simulink model "FireFighter_original"  (R2014a)
settings: Solver=ode45  StartTime=0.0  StopTime=150  RelTol=1e-3
undefined symbols (not defined in the file): DiscIntNeverNeededParam, sigbuilder_block
libraries: simulink x68
(part 1 of 6)
settings Model: NumberOfSteps=200  Creator=rima  LastModifiedBy=rima
settings DataIOCC: InspectSignalLogs=on
settings OptimizationCC: ExpressionDepthLimit=2147483647
settings DebuggingCC: UnderspecifiedInitializationDetection=Classic  SolverPrmCheckMsg=none  StateNameClashWarn=warning

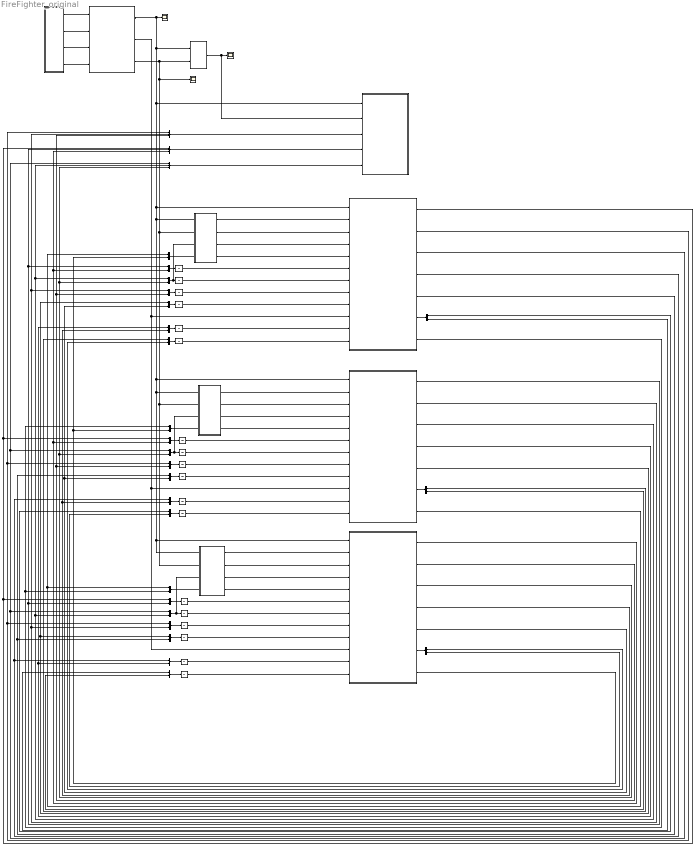
== system FireFighter_original ==
  Demux : Demux  Outputs=2
  Demux1 : Demux  Outputs=2
  Demux2 : Demux  Outputs=2
  FF_Signals : Subsystem
  FF_Signals1 : Subsystem
  FF_Signals2 : Subsystem
  FF_Signals4 : Subsystem
  FireFighter : Stateflow chart  TreatAsAtomicUnit=on
  Helicopter1 : Stateflow chart  TreatAsAtomicUnit=on
  Helicopter2 : Stateflow chart  TreatAsAtomicUnit=on
  Helicopter3 : Stateflow chart  TreatAsAtomicUnit=on
  Inaccuracy : Subsystem
  Leader : Stateflow chart  TreatAsAtomicUnit=on
  Mux{,1,3..7,9..17,20..22,27..28} (21 alike) : Mux  Inputs=2
  Mux18 : Mux  Inputs=3
  Mux19 : Mux  Inputs=3
  Mux2 : Mux  Inputs=3
  Scope1 : Scope
      settings: SaveName=ScopeData10
  Scope11 : Scope
      settings: SaveName=ScopeData37
  Scope2 : Scope
      settings: YMin=-2.5e+12  YMax=2.5e+11  SaveName=ScopeData14
  Unit Delay{,1..14,21..23} (18 alike) : UnitDelay
  wires:
  FF_Signals/1(conn) -> FireFighter/1(ffConn)
  FF_Signals/2(Hconn) -> FireFighter/2(ffHconn)
  Mux2/1 -> Leader/3(HFFPoss)
  Mux1/1 -> FF_Signals1/3(Hpos_inits), Unit Delay2/1
  Mux3/1 -> Unit Delay1/1
  Mux4/1 -> Unit Delay/1
  FireFighter/2(ffMID) -> Helicopter3/10(MID), Helicopter2/10(MID), Helicopter1/10(MID)
  Mux9/1 -> FF_Signals4/3(Hpos_inits), Unit Delay7/1
  Mux10/1 -> Unit Delay6/1
  Mux11/1 -> Unit Delay5/1
  Mux12/1 -> FF_Signals2/3(Hpos_inits), Unit Delay12/1
  Mux13/1 -> Unit Delay11/1
  Mux14/1 -> Unit Delay10/1
  Mux15/1 -> Unit Delay13/1
  Helicopter2/2(HFFPos) -> Mux2/2, Mux17/1, Mux15/2
  Helicopter1/2(HFFPos) -> Mux2/1, Mux16/1, Mux15/1
  Helicopter3/2(HFFPos) -> Mux2/3, Mux17/2, Mux16/2
  Mux16/1 -> Unit Delay8/1
  Mux17/1 -> Unit Delay3/1
  Helicopter1/5(Search_Out) -> Mux11/1, Mux14/2
  Helicopter2/5(Search_Out) -> Mux14/1, Mux4/1
  Helicopter3/5(Search_Out) -> Mux4/2, Mux11/2
  Helicopter3/1(HID) -> Mux18/3, Mux3/2, Mux10/2
  Helicopter1/1(HID) -> Mux18/1, Mux10/1, Mux13/1
  Helicopter2/1(HID) -> Mux18/2, Mux3/1, Mux13/2
  Helicopter2/3(HPos) -> Mux19/2, Mux1/1, Mux12/2
  Helicopter1/3(HPos) -> Mux19/1, Mux9/1, Mux12/1
  Helicopter3/3(HPos) -> Mux19/3, Mux1/2, Mux9/2
  Mux18/1 -> Leader/4(HIDs)
  Mux19/1 -> Leader/5(HPoss)
  Unit Delay5/1 -> Helicopter2/9(Search_In)
  Unit Delay6/1 -> Helicopter2/6(OHIDs)
  Unit Delay7/1 -> Helicopter2/7(OHPoss)
  Unit Delay8/1 -> Helicopter2/8(OHFFPos)
  Unit Delay10/1 -> Helicopter3/9(Search_In)
  Unit Delay11/1 -> Helicopter3/6(OHIDs)
  Unit Delay12/1 -> Helicopter3/7(OHPoss)
  Unit Delay13/1 -> Helicopter3/8(OHFFPos)
  FF_Signals/4(Activate) -> FireFighter/4(ffActivate)
  Mux5/1 -> Unit Delay4/1
  Helicopter3/4(Signal_Out) -> Mux6/2, Mux5/2
  Mux6/1 -> Unit Delay9/1
  Helicopter1/4(Signal_Out) -> Mux6/1, Mux7/1
  Mux7/1 -> Unit Delay14/1
  Helicopter2/4(Signal_Out) -> Mux7/2, Mux5/1
  Unit Delay9/1 -> Helicopter2/11(Signal_In)
  Unit Delay/1 -> Helicopter1/9(Search_In)
  Unit Delay1/1 -> Helicopter1/6(OHIDs)
  Unit Delay2/1 -> Helicopter1/7(OHPoss)
  Unit Delay3/1 -> Helicopter1/8(OHFFPos)
  Unit Delay4/1 -> Helicopter1/11(Signal_In)
  Helicopter1/6(Signal_Reply_Out) -> Demux/1
  Mux/1 -> Unit Delay21/1
  Mux27/1 -> Unit Delay22/1
  Helicopter2/6(Signal_Reply_Out) -> Demux1/1
  Mux28/1 -> Unit Delay23/1
  Helicopter3/6(Signal_Reply_Out) -> Demux2/1
  Demux1/1 -> Mux/1
  Demux2/1 -> Mux/2
  Demux/1 -> Mux27/1
  Demux2/2 -> Mux27/2
  Demux/2 -> Mux28/1
  Demux1/2 -> Mux28/2
  Unit Delay22/1 -> Helicopter2/12(Signal_Reply_In)
  Unit Delay23/1 -> Helicopter3/12(Signal_Reply_In)
  Unit Delay21/1 -> Helicopter1/12(Signal_Reply_In)
  Unit Delay14/1 -> Helicopter3/11(Signal_In)
  FF_Signals/3(FFPos_Out) -> FireFighter/3(ffPos_In)
  FireFighter/3(ffHold) -> Scope11/1, FF_Signals2/2(hold), FF_Signals4/2(hold), FF_Signals1/2(hold), Inaccuracy/2(hold)
  Inaccuracy/1(result) -> Scope2/1, Leader/2(FFPosInacc)
  FF_Signals1/1(HPos_Out) -> Helicopter1/2(HPos_In)
  FF_Signals1/4(SWITCH) -> Helicopter1/5(SWITCH)
  FF_Signals1/2(FFPos_inacc) -> Helicopter1/3(FFPosInacc)
  FireFighter/1(ffPos) -> Scope1/1, Helicopter2/1(FFPos), Helicopter3/1(FFPos), FF_Signals2/1(pos_init), FF_Signals4/1(pos_init), FF_Signals1/1(pos_init), Helicopter1/1(FFPos), Leader/1(FFPos_In), Inaccuracy/1(pos_init)
  FF_Signals4/1(HPos_Out) -> Helicopter2/2(HPos_In)
  FF_Signals4/4(SWITCH) -> Helicopter2/5(SWITCH)
  FF_Signals4/2(FFPos_inacc) -> Helicopter2/3(FFPosInacc)
  FF_Signals2/1(HPos_Out) -> Helicopter3/2(HPos_In)
  FF_Signals2/4(SWITCH) -> Helicopter3/5(SWITCH)
  FF_Signals2/2(FFPos_inacc) -> Helicopter3/3(FFPosInacc)
  FF_Signals1/3(HsInacc) -> Helicopter1/4(HsPosInacc)
  Mux20/1 -> FF_Signals1/4(holds)
  Helicopter2/7(hold) -> Mux20/1, Mux22/1
  Helicopter3/7(hold) -> Mux20/2, Mux21/2
  FF_Signals4/3(HsInacc) -> Helicopter2/4(HsPosInacc)
  Mux21/1 -> FF_Signals4/4(holds)
  Mux22/1 -> FF_Signals2/4(holds)
  Helicopter1/7(hold) -> Mux21/1, Mux22/2
  FF_Signals2/3(HsInacc) -> Helicopter3/4(HsPosInacc)

== system FireFighter_original/FF_Signals ==
  Environment : Subsystem
  FireFighter : Subsystem
  Helicopter Signal : Subsystem  Tag=STV Subsys  LoadFcn=sigbuilder_block('load');  StartFcn=sigbuilder_block('start');  StopFcn=sigbuilder_block('stop');  ClipboardFcn=sigbuilder_block('clipboard');  mask(Sigbuilder block){}
      mask help: Simulink:masks:SigbuilderBlock_MD
      mask init:
      | if ~strcmp(get_param(bdroot(gcbh),'SimulationStatus'),'stopped') tuvar = sigbuilder_block('maskInit'); end
      settings: CopyFcn=sigbuilder_block('copy');  DeleteFcn=sigbuilder_block('delete');  ModelCloseFcn=sigbuilder_block('modelClose');  PreSaveFcn=sigbuilder_block('preSave');  PauseFcn=sigbuilder_block('pause');  ContinueFcn=sigbuilder_block('continue');  NameChangeFcn=sigbuilder_block('namechange');  OpenFcn=sigbuilder_block('open',[451.5 315 606.75 510 ]);  CloseFcn=sigbuilder_block('close');
      mask Display: plot(0, 0, 100, 100,[2, 2, 32, 32, 2], [68, 8, 8, 68, 68],[32, 2], [38, 38], [32, 19, 2],[53, 60, 44], [32, 17, 17, 2],[16, 16, 31, 31]);txt = getActiveGroup(gcbh);text(2, 100, txt,'verticalAlignment', 'top');
  Mux : Mux
  Mux1 : Mux  Inputs=3
  START THE MESSION : Subsystem  Tag=STV Subsys  LoadFcn=sigbuilder_block('load');  StartFcn=sigbuilder_block('start');  StopFcn=sigbuilder_block('stop');  ClipboardFcn=sigbuilder_block('clipboard');  mask(Sigbuilder block){}
      mask help: Simulink:masks:SigbuilderBlock_MD
      mask init:
      | if ~strcmp(get_param(bdroot(gcbh),'SimulationStatus'),'stopped') tuvar = sigbuilder_block('maskInit'); end
      settings: CopyFcn=sigbuilder_block('copy');  DeleteFcn=sigbuilder_block('delete');  ModelCloseFcn=sigbuilder_block('modelClose');  PreSaveFcn=sigbuilder_block('preSave');  PauseFcn=sigbuilder_block('pause');  ContinueFcn=sigbuilder_block('continue');  NameChangeFcn=sigbuilder_block('namechange');  OpenFcn=sigbuilder_block('open',[76.5 537.75 597.75 240 ]);  CloseFcn=sigbuilder_block('close');
      mask Display: plot(0, 0, 100, 100,[2, 2, 32, 32, 2], [68, 8, 8, 68, 68],[32, 2], [38, 38], [32, 19, 2],[53, 60, 44], [32, 17, 17, 2],[16, 16, 31, 31]);txt = getActiveGroup(gcbh);text(2, 100, txt,'verticalAlignment', 'top');
  Scope : Scope
      settings: YMin=1.38778e-17  YMax=0.45  SaveName=ScopeData11
  Scope1 : Scope
      settings: SaveName=ScopeData47
  conn : Outport
  Hconn : Outport  Port=2
  FFPos_Out : Outport  Port=3
  Activate : Outport  Port=4
  wires:
  Environment/1(pos) -> FireFighter/1(pos), Scope/1, FFPos_Out/1
  FireFighter/1(gas) -> Environment/1(gas)
  FireFighter/2(brake) -> Environment/2(brake)
  Helicopter Signal/1(CONN) -> Mux/1, conn/1
  Helicopter Signal/2(HCONN1) -> Mux1/1, Mux/2
  Helicopter Signal/4(HCONN3) -> Mux/4, Mux1/3
  START THE MESSION/1(ACTIVATE) -> Activate/1
  Helicopter Signal/3(HCONN2) -> Mux/3, Mux1/2
  Mux/1 -> Scope1/1
  Mux1/1 -> Hconn/1

== system FireFighter_original/FF_Signals1 ==
  pos_init : Inport
  hold : Inport  Port=2
  Hpos_inits : Inport  Port=3
  holds : Inport  Port=4
  Demux{,1..3} (4 alike) : Demux  Outputs=2
  Environment1 : Subsystem
  FireFighter1 : Subsystem
  Inaccuracy : Subsystem
  Inaccuracy1 : Subsystem
  Inaccuracy2 : Subsystem
  Mux : Mux
  START THE MESSION2 : Subsystem  Tag=STV Subsys  LoadFcn=sigbuilder_block('load');  StartFcn=sigbuilder_block('start');  StopFcn=sigbuilder_block('stop');  ClipboardFcn=sigbuilder_block('clipboard');  mask(Sigbuilder block){}
      mask help: Simulink:masks:SigbuilderBlock_MD
      mask init:
      | if ~strcmp(get_param(bdroot(gcbh),'SimulationStatus'),'stopped') tuvar = sigbuilder_block('maskInit'); end
      settings: CopyFcn=sigbuilder_block('copy');  DeleteFcn=sigbuilder_block('delete');  ModelCloseFcn=sigbuilder_block('modelClose');  PreSaveFcn=sigbuilder_block('preSave');  PauseFcn=sigbuilder_block('pause');  ContinueFcn=sigbuilder_block('continue');  NameChangeFcn=sigbuilder_block('namechange');  OpenFcn=sigbuilder_block('open',[76.5 537.75 597.75 240 ]);  CloseFcn=sigbuilder_block('close');
      mask Display: plot(0, 0, 100, 100,[2, 2, 32, 32, 2], [68, 8, 8, 68, 68],[32, 2], [38, 38], [32, 19, 2],[53, 60, 44], [32, 17, 17, 2],[16, 16, 31, 31]);txt = getActiveGroup(gcbh);text(2, 100, txt,'verticalAlignment', 'top');
  Scope1 : Scope
      settings: YMin=1.38778e-17  YMax=0.45  SaveName=ScopeData4
  HPos_Out : Outport
  FFPos_inacc : Outport  Port=2
  HsInacc : Outport  Port=3
  SWITCH : Outport  Port=4
  wires:
  Environment1/1(pos) -> FireFighter1/1(pos), HPos_Out/1, Scope1/1
  FireFighter1/1(gas) -> Environment1/1(gas)
  FireFighter1/2(brake) -> Environment1/2(brake)
  START THE MESSION2/1(SWITCH) -> SWITCH/1
  Inaccuracy/1(result) -> FFPos_inacc/1
  pos_init/1 -> Inaccuracy/1(pos_init)
  hold/1 -> Inaccuracy/2(hold)
  Inaccuracy1/1(result) -> Demux2/1
  Hpos_inits/1 -> Demux/1
  holds/1 -> Demux1/1
  Demux/1 -> Inaccuracy1/1(Hpos_inits)
  Demux/2 -> Inaccuracy2/1(Hpos_inits)
  Demux1/1 -> Inaccuracy1/2(holds)
  Demux1/2 -> Inaccuracy2/2(holds)
  Inaccuracy2/1(result) -> Demux3/1
  Mux/1 -> HsInacc/1
  Demux2/1 -> Mux/1
  Demux2/2 -> Mux/2
  Demux3/1 -> Mux/3
  Demux3/2 -> Mux/4

== system FireFighter_original/FF_Signals2 ==
  pos_init : Inport
  hold : Inport  Port=2
  Hpos_inits : Inport  Port=3
  holds : Inport  Port=4
  Demux{,1..3} (4 alike) : Demux  Outputs=2
  Environment1 : Subsystem
  FireFighter1 : Subsystem
  Inaccuracy : Subsystem
  Inaccuracy1 : Subsystem
  Inaccuracy2 : Subsystem
  Mux : Mux
  START THE MESSION2 : Subsystem  Tag=STV Subsys  LoadFcn=sigbuilder_block('load');  StartFcn=sigbuilder_block('start');  StopFcn=sigbuilder_block('stop');  ClipboardFcn=sigbuilder_block('clipboard');  mask(Sigbuilder block){}
      mask help: Simulink:masks:SigbuilderBlock_MD
      mask init:
      | if ~strcmp(get_param(bdroot(gcbh),'SimulationStatus'),'stopped') tuvar = sigbuilder_block('maskInit'); end
      settings: CopyFcn=sigbuilder_block('copy');  DeleteFcn=sigbuilder_block('delete');  ModelCloseFcn=sigbuilder_block('modelClose');  PreSaveFcn=sigbuilder_block('preSave');  PauseFcn=sigbuilder_block('pause');  ContinueFcn=sigbuilder_block('continue');  NameChangeFcn=sigbuilder_block('namechange');  OpenFcn=sigbuilder_block('open',[76.5 537.75 597.75 240 ]);  CloseFcn=sigbuilder_block('close');
      mask Display: plot(0, 0, 100, 100,[2, 2, 32, 32, 2], [68, 8, 8, 68, 68],[32, 2], [38, 38], [32, 19, 2],[53, 60, 44], [32, 17, 17, 2],[16, 16, 31, 31]);txt = getActiveGroup(gcbh);text(2, 100, txt,'verticalAlignment', 'top');
  Scope1 : Scope
      settings: YMin=1.38778e-17  YMax=0.45  SaveName=ScopeData4
  HPos_Out : Outport
  FFPos_inacc : Outport  Port=2
  HsInacc : Outport  Port=3
  SWITCH : Outport  Port=4
  wires:
  Environment1/1(pos) -> FireFighter1/1(pos), HPos_Out/1, Scope1/1
  FireFighter1/1(gas) -> Environment1/1(gas)
  FireFighter1/2(brake) -> Environment1/2(brake)
  START THE MESSION2/1(SWITCH) -> SWITCH/1
  Inaccuracy/1(result) -> FFPos_inacc/1
  pos_init/1 -> Inaccuracy/1(pos_init)
  hold/1 -> Inaccuracy/2(hold)
  Inaccuracy1/1(result) -> Demux2/1
  Hpos_inits/1 -> Demux/1
  holds/1 -> Demux1/1
  Demux/1 -> Inaccuracy1/1(Hpos_inits)
  Demux/2 -> Inaccuracy2/1(Hpos_inits)
  Demux1/1 -> Inaccuracy1/2(holds)
  Demux1/2 -> Inaccuracy2/2(holds)
  Inaccuracy2/1(result) -> Demux3/1
  Mux/1 -> HsInacc/1
  Demux2/1 -> Mux/1
  Demux2/2 -> Mux/2
  Demux3/1 -> Mux/3
  Demux3/2 -> Mux/4

== system FireFighter_original/FF_Signals4 ==
  pos_init : Inport
  hold : Inport  Port=2
  Hpos_inits : Inport  Port=3
  holds : Inport  Port=4
  Demux{,1..3} (4 alike) : Demux  Outputs=2
  Environment1 : Subsystem
  FireFighter1 : Subsystem
  Inaccuracy : Subsystem
  Inaccuracy1 : Subsystem
  Inaccuracy2 : Subsystem
  Mux : Mux
  START THE MESSION2 : Subsystem  Tag=STV Subsys  LoadFcn=sigbuilder_block('load');  StartFcn=sigbuilder_block('start');  StopFcn=sigbuilder_block('stop');  ClipboardFcn=sigbuilder_block('clipboard');  mask(Sigbuilder block){}
      mask help: Simulink:masks:SigbuilderBlock_MD
      mask init:
      | if ~strcmp(get_param(bdroot(gcbh),'SimulationStatus'),'stopped') tuvar = sigbuilder_block('maskInit'); end
      settings: CopyFcn=sigbuilder_block('copy');  DeleteFcn=sigbuilder_block('delete');  ModelCloseFcn=sigbuilder_block('modelClose');  PreSaveFcn=sigbuilder_block('preSave');  PauseFcn=sigbuilder_block('pause');  ContinueFcn=sigbuilder_block('continue');  NameChangeFcn=sigbuilder_block('namechange');  OpenFcn=sigbuilder_block('open',[76.5 537.75 597.75 240 ]);  CloseFcn=sigbuilder_block('close');
      mask Display: plot(0, 0, 100, 100,[2, 2, 32, 32, 2], [68, 8, 8, 68, 68],[32, 2], [38, 38], [32, 19, 2],[53, 60, 44], [32, 17, 17, 2],[16, 16, 31, 31]);txt = getActiveGroup(gcbh);text(2, 100, txt,'verticalAlignment', 'top');
  Scope1 : Scope
      settings: YMin=1.38778e-17  YMax=0.45  SaveName=ScopeData4
  HPos_Out : Outport
  FFPos_inacc : Outport  Port=2
  HsInacc : Outport  Port=3
  SWITCH : Outport  Port=4
  wires:
  Environment1/1(pos) -> FireFighter1/1(pos), HPos_Out/1, Scope1/1
  FireFighter1/1(gas) -> Environment1/1(gas)
  FireFighter1/2(brake) -> Environment1/2(brake)
  START THE MESSION2/1(SWITCH) -> SWITCH/1
  Inaccuracy/1(result) -> FFPos_inacc/1
  pos_init/1 -> Inaccuracy/1(pos_init)
  hold/1 -> Inaccuracy/2(hold)
  Inaccuracy1/1(result) -> Demux2/1
  Hpos_inits/1 -> Demux/1
  holds/1 -> Demux1/1
  Demux/1 -> Inaccuracy1/1(Hpos_inits)
  Demux/2 -> Inaccuracy2/1(Hpos_inits)
  Demux1/1 -> Inaccuracy1/2(holds)
  Demux1/2 -> Inaccuracy2/2(holds)
  Inaccuracy2/1(result) -> Demux3/1
  Mux/1 -> HsInacc/1
  Demux2/1 -> Mux/1
  Demux2/2 -> Mux/2
  Demux3/1 -> Mux/3
  Demux3/2 -> Mux/4

== system FireFighter_original/Inaccuracy ==
  note: max
  pos_init : Inport
  hold : Inport  Port=2
  Mux29 : Mux  Inputs=2
  Product : Product
  Product1 : Product
  Scope{1..3,5..7,9} (7 alike) : Scope
      Scope1 settings: SaveName=ScopeData29
      Scope2 settings: SaveName=ScopeData43
      Scope3 settings: SaveName=ScopeData35
      Scope5 settings: SaveName=ScopeData46
      Scope6 settings: SaveName=ScopeData48
      Scope7 settings: TimeRange=150  SaveName=ScopeData57
      Scope9 settings: SaveName=ScopeData44
  Subsystem1 : Subsystem
  Subsystem2 : Subsystem
  Subtract1 : Sum  Inputs=-+
  Unit Delay1 : UnitDelay  SampleTime=10
  result : Outport
  wires:
  Subsystem2/1(min) -> Product/1, Scope2/1  "min"
  pos_init/1 -> Subsystem1/1(pos_init), Subsystem2/1(pos_init), Scope1/1
  Mux29/1 -> result/1
  Subsystem1/1(max) -> Product1/2, Scope9/1
  Product/1 -> Mux29/1, Scope6/1, Subtract1/1
  Product1/1 -> Scope5/1, Mux29/2, Subtract1/2
  hold/1 -> Subsystem2/2(hold), Scope3/1, Product/2, Product1/1, Subsystem1/2(hold)
  Subtract1/1 -> Scope7/1

== system FireFighter_original/FF_Signals/Environment ==
  note: F_hill
  note: F_eng_resistance
  note: F_resistance
  note: F_eng
  note: position
  note: speed
  note: slope
  gas : Inport
  brake : Inport  Port=2
  1/mass2 : Gain  Gain=0.001
  Discrete-Time Integrator : DiscreteIntegrator  SampleTime=-1  ICPrevOutput=DiscIntNeverNeededParam  ICPrevScaledInput=DiscIntNeverNeededParam
  Discrete-Time Integrator1 : DiscreteIntegrator  SampleTime=-1  ICPrevOutput=DiscIntNeverNeededParam  ICPrevScaledInput=DiscIntNeverNeededParam
  Fast - to - Slow : RateTransition  OutPortSampleTimeMultiple=0.05  OutPortSampleTime=0.1
  "Fast - to - Slow1 " : RateTransition  OutPortSampleTimeMultiple=0.05  OutPortSampleTime=0.1
  Fcn : Fcn  Expr=u(1)/0.005
  Gain1 : Gain  Gain=0.0005
  Max Torque by rpm6 : Lookup_n-D  NumberOfTableDimensions=1  BreakpointsForDimension1=[0;8;20;28;40;60;80;100;120;140;160;180;200]  Table=[165;180;180;170;170;150;115;97;80;70;60;50;40]  RndMeth=Simplest  InputSameDT=on
  Max Torque by rpm9 : Lookup_n-D  NumberOfTableDimensions=1  BreakpointsForDimension1=[0:1000:15000]  Table=[0;pi/60;pi/30;pi/20;pi/15;pi/12;0;0;-pi/18;-pi/36;0;0;0;0;0;0]  RndMeth=Simplest  InputSameDT=on
  Product1 : Product  RndMeth=Zero
  Scope{2..3,6..15,27} (13 alike) : Scope
      Scope10 settings: SaveName=ScopeData23
      Scope11 settings: TimeRange=10  YMin=-50  YMax=300  SaveName=ScopeData26
      Scope12 settings: SaveName=ScopeData32
      Scope13 settings: SaveName=ScopeData33
      Scope14 settings: SaveName=ScopeData15
      Scope15 settings: SaveName=ScopeData19
      Scope2 settings: TimeRange=10  YMin=-50  YMax=300  SaveName=ScopeData6
      Scope27 settings: TimeRange=10  YMin=-50  YMax=300  SaveName=ScopeData49
      Scope3 settings: SaveName=ScopeData8
      Scope6 settings: TimeRange=100  YMin=89.9904  YMax=89.9913  SaveName=ScopeData16
      Scope7 settings: SaveName=ScopeData10
      Scope8 settings: SaveName=ScopeData21
      Scope9 settings: SaveName=ScopeData22
  Slow - to - Fast : RateTransition  OutPortSampleTimeMultiple=0.05  OutPortSampleTime=0.05
  Step1 : Step  Time=0  After=60
  Sum1 : Sum  Inputs=|++
  Sum4 : Sum  Inputs=|+---
  Trigonometric Function1 : Trigonometry
  brake force1 : Gain  Gain=10000
  g1 : Gain  Gain=9.80665
  mass3 : Gain  Gain=1000
  pos : Outport
  wires:
  Step1/1 -> Sum1/2
  Product1/1 -> Fcn/1
  brake force1/1 -> Scope12/1, Sum4/2
  Sum4/1 -> Scope7/1, 1/mass2/1
  1/mass2/1 -> Discrete-Time Integrator/1, Scope8/1
  Gain1/1 -> Scope13/1, Sum4/3
  gas/1 -> Scope14/1, Fast - to - Slow/1
  brake/1 -> Scope15/1, "Fast - to - Slow1 "/1
  Discrete-Time Integrator/1 -> Max Torque by rpm6/1, Gain1/1, Discrete-Time Integrator1/1, Scope6/1
  Discrete-Time Integrator1/1 -> Max Torque by rpm9/1, Scope2/1, Sum1/1
  Max Torque by rpm9/1 -> Trigonometric Function1/1
  g1/1 -> mass3/1
  Trigonometric Function1/1 -> g1/1
  mass3/1 -> Sum4/4, Scope3/1
  Fcn/1 -> Scope10/1, Sum4/1
  Fast - to - Slow/1 -> Product1/2
  "Fast - to - Slow1 "/1 -> brake force1/1
  Sum1/1 -> Scope27/1, Slow - to - Fast/1
  Slow - to - Fast/1 -> pos/1, Scope11/1
  Max Torque by rpm6/1 -> Product1/1, Scope9/1

== system FireFighter_original/FF_Signals/FireFighter ==
  note: current speed
  note: speed=90
  pos : Inport
  Constant : Constant  Value=0
  Constant2 : Constant  Value=140
  Discrete Derivative : simulink/Discrete/Discrete Derivative  gainval=1.0  ICPrevScaledInput=0.0  InputProcessing=Inherited  OutMin=[]  OutMax=[]  OutDataType=fixdt(1, 16)  OutScaling=2^-10  DoSatur=off
  Discrete PID Controller : simulink/Continuous/PID Controller  Controller=PI  TimeDomain=Discrete-time  SampleTime=-1  IntegratorMethod=Forward Euler  FilterMethod=Forward Euler  Form=Parallel  P=0.05  I=0.000228325  D=0  N=100  InitialConditionSource=internal  InitialConditionForIntegrator=0  InitialConditionForFilter=0  ExternalReset=none  LimitOutput=on  UpperSaturationLimit=1  LowerSaturationLimit=-1  LinearizeAsGain=off  AntiWindupMode=back-calculation  Kb=0.01  TrackingMode=off  Kt=1  PParamMin=[]  PParamMax=[]  IParamMin=[]  IParamMax=[]  DParamMin=[]  DParamMax=[]  NParamMin=[]  NParamMax=[]  KbParamMin=[]  KbParamMax=[]  KtParamMin=[]  KtParamMax=[]  POutMin=[]  POutMax=[]  IOutMin=[]  IOutMax=[]  DOutMin=[]  DOutMax=[]  NOutMin=[]  NOutMax=[]  KbOutMin=[]  KbOutMax=[]  KtOutMin=[]  KtOutMax=[]  IntegratorOutMin=[]  IntegratorOutMax=[]  FilterOutMin=[]  FilterOutMax=[]  SumOutMin=[]  SumOutMax=[]  SumI1OutMin=[]  SumI1OutMax=[]  SumI2OutMin=[]  SumI2OutMax=[]  SumI3OutMin=[]  SumI3OutMax=[]  SumDOutMin=[]  SumDOutMax=[]  SaturationOutMin=[]  SaturationOutMax=[]  IntegratorContinuousStateAttributes=''  IntegratorStateMustResolveToSignalObject=off  IntegratorRTWStateStorageClass=Auto  FilterContinuousStateAttributes=''  FilterStateMustResolveToSignalObject=off  FilterRTWStateStorageClass=Auto
  Fast - to -Slow : RateTransition  OutPortSampleTimeMultiple=0.05  OutPortSampleTime=0.1
  Gain : Gain  Gain=50
  Gain1 : Gain  Gain=-1
  Scope{1..2,4..9,11..13} (11 alike) : Scope
      Scope1 settings: TimeRange=100  YMin=90  YMax=130
      Scope11 settings: YMin=-300  YMax=300  SaveName=ScopeData28
      Scope12 settings: YMin=-300  YMax=300  SaveName=ScopeData30
      Scope13 settings: SaveName=ScopeData31
      Scope2 settings: YMin=-300  YMax=300  SaveName=ScopeData2
      Scope4 settings: YMin=-300  YMax=300  SaveName=ScopeData17
      Scope5 settings: SaveName=ScopeData20
      Scope6 settings: YMin=-300  YMax=300  SaveName=ScopeData18
      Scope7 settings: YMin=-300  YMax=300  SaveName=ScopeData24
      Scope8 settings: TimeRange=10  SaveName=ScopeData25
      Scope9 settings: SaveName=ScopeData38
  Signal Builder : Subsystem  Tag=STV Subsys  LoadFcn=sigbuilder_block('load');  StartFcn=sigbuilder_block('start');  StopFcn=sigbuilder_block('stop');  ClipboardFcn=sigbuilder_block('clipboard');  mask(Sigbuilder block){}
      mask help: Simulink:masks:SigbuilderBlock_MD
      mask init:
      | if ~strcmp(get_param(bdroot(gcbh),'SimulationStatus'),'stopped') tuvar = sigbuilder_block('maskInit'); end
      settings: CopyFcn=sigbuilder_block('copy');  DeleteFcn=sigbuilder_block('delete');  ModelCloseFcn=sigbuilder_block('modelClose');  PreSaveFcn=sigbuilder_block('preSave');  PauseFcn=sigbuilder_block('pause');  ContinueFcn=sigbuilder_block('continue');  NameChangeFcn=sigbuilder_block('namechange');  OpenFcn=sigbuilder_block('open',[359.25 300.75 550.5 399.75 ]);  CloseFcn=sigbuilder_block('close');
      mask Display: plot(0, 0, 100, 100,[2, 2, 32, 32, 2], [68, 8, 8, 68, 68],[32, 2], [38, 38], [32, 19, 2],[53, 60, 44], [32, 17, 17, 2],[16, 16, 31, 31]);txt = getActiveGroup(gcbh);text(2, 100, txt,'verticalAlignment', 'top');
  Slow - to - Fast : RateTransition  OutPortSampleTimeMultiple=0.05  OutPortSampleTime=0.05
  Slow - to - Fast1 : RateTransition  OutPortSampleTimeMultiple=0.05  OutPortSampleTime=0.05
  Sum : Sum  Inputs=|+-
  Sum1 : Sum  Inputs=|++
  Switch : Switch
  Switch1 : Switch
  Zero-Order Hold : ZeroOrderHold  SampleTime=0.1
  gas : Outport
  brake : Outport  Port=2
  wires:
  Discrete Derivative/1 -> Scope8/1, Sum/2
  Signal Builder/1(Signal 1) -> Gain/1
  Gain/1 -> Zero-Order Hold/1
  Constant2/1 -> Sum1/2
  Discrete PID Controller/1 -> Scope2/1, Scope7/1, Switch/1, Switch/2, Switch1/2, Gain1/1
  Gain1/1 -> Switch1/3
  Switch/1 -> Slow - to - Fast/1, Scope4/1
  Constant/1 -> Switch/3, Switch1/1
  Switch1/1 -> Slow - to - Fast1/1, Scope6/1
  pos/1 -> Scope13/1, Fast - to -Slow/1
  Sum/1 -> Discrete PID Controller/1, Scope9/1
  Fast - to -Slow/1 -> Discrete Derivative/1, Scope5/1
  Slow - to - Fast/1 -> Scope11/1, gas/1
  Slow - to - Fast1/1 -> Scope12/1, brake/1
  Sum1/1 -> Scope1/1, Sum/1
  Zero-Order Hold/1 -> Sum1/1

== system FireFighter_original/FF_Signals/Helicopter Signal ==
  Demux : Demux  Tag=STV Demux
  FromWs : FromWorkspace  Tag=STV FromWs  VariableName=tuvar  SampleTime=0
      SigBuilderData=|
      | common.afterFinalStr = 'Extrapolate'
      | common.sampleTime = 0
      | dataSet.timeRange = [0 150]
      | dataSet.name = 'Group 1'
      | sbobj.Groups.Name = 'Group 1'
      | sbobj.Groups.Signals(1).Name = 'CONN'
      | sbobj.Groups.Signals(1).XData = [0 7 7 14 14 130 130 150]
      | sbobj.Groups.Signals(1).YData = [0 0 1 1 0 0 1 1]
      | sbobj.Groups.Signals(2).Name = 'HCONN1'
      | sbobj.Groups.Signals(2).XData = [0 25 25 32 32 150]
      | sbobj.Groups.Signals(2).YData = [0 0 1 1 0 0]
      | sbobj.Groups.Signals(3).Name = 'HCONN2'
      | sbobj.Groups.Signals(3).XData = [0 60 60 64 64 150]
      | sbobj.Groups.Signals(3).YData = [0 0 1 1 0 0]
      | sbobj.Groups.Signals(4).Name = 'HCONN3'
      | sbobj.Groups.Signals(4).XData = [0 65 65 68 68 150]
      | sbobj.Groups.Signals(4).YData = [0 0 1 1 0 0]
      | sbobj.Groups.TimeRange = [0 150]
  CONN : Outport  Tag=STV Outport
  HCONN1 : Outport  Tag=STV Outport  Port=2
  HCONN2 : Outport  Tag=STV Outport  Port=3
  HCONN3 : Outport  Tag=STV Outport  Port=4
  wires:
  FromWs/1 -> Demux/1
  Demux/1 -> CONN/1
  Demux/2 -> HCONN1/1
  Demux/3 -> HCONN2/1
  Demux/4 -> HCONN3/1

== system FireFighter_original/FF_Signals/START THE MESSION ==
  Demux : Demux  Tag=STV Demux  Outputs=1
  FromWs : FromWorkspace  Tag=STV FromWs  VariableName=tuvar  SampleTime=0
      SigBuilderData=|
      | common.afterFinalStr = 'Extrapolate'
      | common.sampleTime = 0
      | dataSet.timeRange = [0 150]
      | dataSet.name = 'Group 1'
      | sbobj.Groups.Name = 'Group 1'
      | sbobj.Groups.Signals.Name = 'ACTIVATE'
      | sbobj.Groups.Signals.XData = [0 2 2 150]
      | sbobj.Groups.Signals.YData = [0 0 1 1]
      | sbobj.Groups.TimeRange = [0 150]
  ACTIVATE : Outport  Tag=STV Outport
  wires:
  FromWs/1 -> Demux/1
  Demux/1 -> ACTIVATE/1

== system FireFighter_original/FF_Signals1/Environment1 ==
  note: F_hill
  note: F_eng_resistance
  note: F_resistance
  note: F_eng
  note: position
  note: speed
  note: slope
  gas : Inport
  brake : Inport  Port=2
  1/mass2 : Gain  Gain=0.001
  Discrete-Time Integrator : DiscreteIntegrator  SampleTime=-1  ICPrevOutput=DiscIntNeverNeededParam  ICPrevScaledInput=DiscIntNeverNeededParam
  Discrete-Time Integrator1 : DiscreteIntegrator  SampleTime=-1  ICPrevOutput=DiscIntNeverNeededParam  ICPrevScaledInput=DiscIntNeverNeededParam
  Fast - to - Slow : RateTransition  OutPortSampleTimeMultiple=0.05  OutPortSampleTime=0.1
  "Fast - to - Slow1 " : RateTransition  OutPortSampleTimeMultiple=0.05  OutPortSampleTime=0.1
  Fcn : Fcn  Expr=u(1)/0.005
  Gain1 : Gain  Gain=0.0005
  Max Torque by rpm6 : Lookup_n-D  NumberOfTableDimensions=1  BreakpointsForDimension1=[0;8;20;28;40;60;80;100;120;140;160;180;200]  Table=[165;180;180;170;170;150;115;97;80;70;60;50;40]  RndMeth=Simplest  InputSameDT=on
  Max Torque by rpm9 : Lookup_n-D  NumberOfTableDimensions=1  BreakpointsForDimension1=[0:1000:15000]  Table=[0;pi/60;pi/30;pi/20;pi/15;pi/12;0;0;-pi/18;-pi/36;0;0;0;0;0;0]  RndMeth=Simplest  InputSameDT=on
  Product1 : Product  RndMeth=Zero
  Scope{2..3,6..15,27} (13 alike) : Scope
      Scope10 settings: SaveName=ScopeData23
      Scope11 settings: TimeRange=10  YMin=-50  YMax=300  SaveName=ScopeData26
      Scope12 settings: SaveName=ScopeData32
      Scope13 settings: SaveName=ScopeData33
      Scope14 settings: SaveName=ScopeData15
      Scope15 settings: SaveName=ScopeData19
      Scope2 settings: TimeRange=10  YMin=-50  YMax=300  SaveName=ScopeData6
      Scope27 settings: TimeRange=10  YMin=-50  YMax=300  SaveName=ScopeData49
      Scope3 settings: SaveName=ScopeData8
      Scope6 settings: TimeRange=100  YMin=89.9904  YMax=89.9913  SaveName=ScopeData16
      Scope7 settings: SaveName=ScopeData10
      Scope8 settings: SaveName=ScopeData21
      Scope9 settings: SaveName=ScopeData22
  Slow - to - Fast : RateTransition  OutPortSampleTimeMultiple=0.05  OutPortSampleTime=0.05
  Step1 : Step  Time=0  After=60
  Sum1 : Sum  Inputs=|++
  Sum4 : Sum  Inputs=|+---
  Trigonometric Function1 : Trigonometry
  brake force1 : Gain  Gain=10000
  g1 : Gain  Gain=9.80665
  mass3 : Gain  Gain=1000
  pos : Outport
  wires:
  Step1/1 -> Sum1/2
  Product1/1 -> Fcn/1
  brake force1/1 -> Scope12/1, Sum4/2
  Sum4/1 -> Scope7/1, 1/mass2/1
  1/mass2/1 -> Discrete-Time Integrator/1, Scope8/1
  Gain1/1 -> Scope13/1, Sum4/3
  gas/1 -> Scope14/1, Fast - to - Slow/1
  brake/1 -> Scope15/1, "Fast - to - Slow1 "/1
  Discrete-Time Integrator/1 -> Max Torque by rpm6/1, Gain1/1, Discrete-Time Integrator1/1, Scope6/1
  Discrete-Time Integrator1/1 -> Max Torque by rpm9/1, Scope2/1, Sum1/1
  Max Torque by rpm9/1 -> Trigonometric Function1/1
  g1/1 -> mass3/1
  Trigonometric Function1/1 -> g1/1
  mass3/1 -> Sum4/4, Scope3/1
  Fcn/1 -> Scope10/1, Sum4/1
  Fast - to - Slow/1 -> Product1/2
  "Fast - to - Slow1 "/1 -> brake force1/1
  Sum1/1 -> Scope27/1, Slow - to - Fast/1
  Slow - to - Fast/1 -> pos/1, Scope11/1
  Max Torque by rpm6/1 -> Product1/1, Scope9/1

== system FireFighter_original/FF_Signals1/FireFighter1 ==
  note: current speed
  note: speed=90
  pos : Inport
  Constant : Constant  Value=0
  Constant2 : Constant  Value=90
  Discrete Derivative : simulink/Discrete/Discrete Derivative  gainval=1.0  ICPrevScaledInput=0.0  InputProcessing=Inherited  OutMin=[]  OutMax=[]  OutDataType=fixdt(1, 16)  OutScaling=2^-10  DoSatur=off
  Discrete PID Controller : simulink/Continuous/PID Controller  Controller=PI  TimeDomain=Discrete-time  SampleTime=-1  IntegratorMethod=Forward Euler  FilterMethod=Forward Euler  Form=Parallel  P=0.05  I=0.000228325  D=0  N=100  InitialConditionSource=internal  InitialConditionForIntegrator=0  InitialConditionForFilter=0  ExternalReset=none  LimitOutput=on  UpperSaturationLimit=1  LowerSaturationLimit=-1  LinearizeAsGain=off  AntiWindupMode=back-calculation  Kb=0.01  TrackingMode=off  Kt=1  PParamMin=[]  PParamMax=[]  IParamMin=[]  IParamMax=[]  DParamMin=[]  DParamMax=[]  NParamMin=[]  NParamMax=[]  KbParamMin=[]  KbParamMax=[]  KtParamMin=[]  KtParamMax=[]  POutMin=[]  POutMax=[]  IOutMin=[]  IOutMax=[]  DOutMin=[]  DOutMax=[]  NOutMin=[]  NOutMax=[]  KbOutMin=[]  KbOutMax=[]  KtOutMin=[]  KtOutMax=[]  IntegratorOutMin=[]  IntegratorOutMax=[]  FilterOutMin=[]  FilterOutMax=[]  SumOutMin=[]  SumOutMax=[]  SumI1OutMin=[]  SumI1OutMax=[]  SumI2OutMin=[]  SumI2OutMax=[]  SumI3OutMin=[]  SumI3OutMax=[]  SumDOutMin=[]  SumDOutMax=[]  SaturationOutMin=[]  SaturationOutMax=[]  IntegratorContinuousStateAttributes=''  IntegratorStateMustResolveToSignalObject=off  IntegratorRTWStateStorageClass=Auto  FilterContinuousStateAttributes=''  FilterStateMustResolveToSignalObject=off  FilterRTWStateStorageClass=Auto
  Fast - to -Slow : RateTransition  OutPortSampleTimeMultiple=0.05  OutPortSampleTime=0.1
  Gain : Gain  Gain=50
  Gain1 : Gain  Gain=-1
  Scope{1..2,4..9,11..13} (11 alike) : Scope
      Scope1 settings: TimeRange=100  YMin=90  YMax=130
      Scope11 settings: YMin=-300  YMax=300  SaveName=ScopeData28
      Scope12 settings: YMin=-300  YMax=300  SaveName=ScopeData30
      Scope13 settings: SaveName=ScopeData31
      Scope2 settings: YMin=-300  YMax=300  SaveName=ScopeData2
      Scope4 settings: YMin=-300  YMax=300  SaveName=ScopeData17
      Scope5 settings: SaveName=ScopeData20
      Scope6 settings: YMin=-300  YMax=300  SaveName=ScopeData18
      Scope7 settings: YMin=-300  YMax=300  SaveName=ScopeData24
      Scope8 settings: TimeRange=10  SaveName=ScopeData25
      Scope9 settings: SaveName=ScopeData38
  Signal Builder : Subsystem  Tag=STV Subsys  LoadFcn=sigbuilder_block('load');  StartFcn=sigbuilder_block('start');  StopFcn=sigbuilder_block('stop');  ClipboardFcn=sigbuilder_block('clipboard');  mask(Sigbuilder block){}
      mask help: Simulink:masks:SigbuilderBlock_MD
      mask init:
      | if ~strcmp(get_param(bdroot(gcbh),'SimulationStatus'),'stopped') tuvar = sigbuilder_block('maskInit'); end
      settings: CopyFcn=sigbuilder_block('copy');  DeleteFcn=sigbuilder_block('delete');  ModelCloseFcn=sigbuilder_block('modelClose');  PreSaveFcn=sigbuilder_block('preSave');  PauseFcn=sigbuilder_block('pause');  ContinueFcn=sigbuilder_block('continue');  NameChangeFcn=sigbuilder_block('namechange');  OpenFcn=sigbuilder_block('open',[359.25 300.75 550.5 399.75 ]);  CloseFcn=sigbuilder_block('close');
      mask Display: plot(0, 0, 100, 100,[2, 2, 32, 32, 2], [68, 8, 8, 68, 68],[32, 2], [38, 38], [32, 19, 2],[53, 60, 44], [32, 17, 17, 2],[16, 16, 31, 31]);txt = getActiveGroup(gcbh);text(2, 100, txt,'verticalAlignment', 'top');
  Slow - to - Fast : RateTransition  OutPortSampleTimeMultiple=0.05  OutPortSampleTime=0.05
  Slow - to - Fast1 : RateTransition  OutPortSampleTimeMultiple=0.05  OutPortSampleTime=0.05
  Sum : Sum  Inputs=|+-
  Sum1 : Sum  Inputs=|++
  Switch : Switch
  Switch1 : Switch
  Zero-Order Hold : ZeroOrderHold  SampleTime=0.1
  gas : Outport
  brake : Outport  Port=2
  wires:
  Discrete Derivative/1 -> Scope8/1, Sum/2
  Signal Builder/1(Signal 1) -> Gain/1
  Gain/1 -> Zero-Order Hold/1
  Constant2/1 -> Sum1/2
  Discrete PID Controller/1 -> Scope2/1, Scope7/1, Switch/1, Switch/2, Switch1/2, Gain1/1
  Gain1/1 -> Switch1/3
  Switch/1 -> Slow - to - Fast/1, Scope4/1
  Constant/1 -> Switch/3, Switch1/1
  Switch1/1 -> Slow - to - Fast1/1, Scope6/1
  pos/1 -> Scope13/1, Fast - to -Slow/1
  Sum/1 -> Discrete PID Controller/1, Scope9/1
  Fast - to -Slow/1 -> Discrete Derivative/1, Scope5/1
  Slow - to - Fast/1 -> Scope11/1, gas/1
  Slow - to - Fast1/1 -> Scope12/1, brake/1
  Sum1/1 -> Scope1/1, Sum/1
  Zero-Order Hold/1 -> Sum1/1

== system FireFighter_original/FF_Signals1/Inaccuracy ==
  note: max
  pos_init : Inport
  hold : Inport  Port=2
  Mux29 : Mux  Inputs=2
  Product : Product
  Product1 : Product
  Scope{1..3,5..7,9} (7 alike) : Scope
      Scope1 settings: SaveName=ScopeData29
      Scope2 settings: SaveName=ScopeData43
      Scope3 settings: SaveName=ScopeData35
      Scope5 settings: SaveName=ScopeData46
      Scope6 settings: SaveName=ScopeData48
      Scope7 settings: TimeRange=150  SaveName=ScopeData57
      Scope9 settings: SaveName=ScopeData44
  Subsystem1 : Subsystem
  Subsystem2 : Subsystem
  Subtract1 : Sum  Inputs=-+
  result : Outport
  wires:
  Subsystem2/1(min) -> Product/1, Scope2/1  "min"
  pos_init/1 -> Subsystem1/1(pos_init), Subsystem2/1(pos_init), Scope1/1
  Mux29/1 -> result/1
  Subsystem1/1(max) -> Product1/2, Scope9/1
  Product/1 -> Mux29/1, Scope6/1, Subtract1/1
  Product1/1 -> Scope5/1, Mux29/2, Subtract1/2
  hold/1 -> Subsystem2/2(hold), Scope3/1, Product/2, Product1/1, Subsystem1/2(hold)
  Subtract1/1 -> Scope7/1

== system FireFighter_original/FF_Signals1/Inaccuracy1 ==
  note: max
  Hpos_inits : Inport
  holds : Inport  Port=2
  Mux29 : Mux  Inputs=2
  Product : Product
  Product1 : Product
  Scope{1..3,5..7,9} (7 alike) : Scope
      Scope1 settings: SaveName=ScopeData29
      Scope2 settings: SaveName=ScopeData43
      Scope3 settings: SaveName=ScopeData35
      Scope5 settings: SaveName=ScopeData46
      Scope6 settings: SaveName=ScopeData48
      Scope7 settings: TimeRange=150  SaveName=ScopeData57
      Scope9 settings: SaveName=ScopeData44
  Subsystem1 : Subsystem
  Subsystem2 : Subsystem
  Subtract1 : Sum  Inputs=-+
  result : Outport
  wires:
  Subsystem2/1(min) -> Product/1, Scope2/1  "min"
  Hpos_inits/1 -> Subsystem1/1(pos_init), Subsystem2/1(pos_init), Scope1/1
  Mux29/1 -> result/1
  Subsystem1/1(max) -> Product1/2, Scope9/1
  Product/1 -> Mux29/1, Scope6/1, Subtract1/1
  Product1/1 -> Scope5/1, Mux29/2, Subtract1/2
  holds/1 -> Subsystem2/2(hold), Scope3/1, Product/2, Product1/1, Subsystem1/2(hold)
  Subtract1/1 -> Scope7/1

== system FireFighter_original/FF_Signals1/Inaccuracy2 ==
  note: max
  Hpos_inits : Inport
  holds : Inport  Port=2
  Mux29 : Mux  Inputs=2
  Product : Product
  Product1 : Product
  Scope{1..3,5..7,9} (7 alike) : Scope
      Scope1 settings: SaveName=ScopeData29
      Scope2 settings: SaveName=ScopeData43
      Scope3 settings: SaveName=ScopeData35
      Scope5 settings: SaveName=ScopeData46
      Scope6 settings: SaveName=ScopeData48
      Scope7 settings: TimeRange=150  SaveName=ScopeData57
      Scope9 settings: SaveName=ScopeData44
  Subsystem1 : Subsystem
  Subsystem2 : Subsystem
  Subtract1 : Sum  Inputs=-+
  result : Outport
  wires:
  Subsystem2/1(min) -> Product/1, Scope2/1  "min"
  Hpos_inits/1 -> Subsystem1/1(pos_init), Subsystem2/1(pos_init), Scope1/1
  Mux29/1 -> result/1
  Subsystem1/1(max) -> Product1/2, Scope9/1
  Product/1 -> Mux29/1, Scope6/1, Subtract1/1
  Product1/1 -> Scope5/1, Mux29/2, Subtract1/2
  holds/1 -> Subsystem2/2(hold), Scope3/1, Product/2, Product1/1, Subsystem1/2(hold)
  Subtract1/1 -> Scope7/1

== system FireFighter_original/FF_Signals1/START THE MESSION2 ==
  Demux : Demux  Tag=STV Demux  Outputs=1
  FromWs : FromWorkspace  Tag=STV FromWs  VariableName=tuvar  SampleTime=0
      SigBuilderData=|
      | common.afterFinalStr = 'Extrapolate'
      | common.sampleTime = 0
      | dataSet.timeRange = [0 1000]
      | dataSet.name = 'Group 1'
      | sbobj.Groups.Name = 'Group 1'
      | sbobj.Groups.Signals.Name = 'SWITCH'
      | sbobj.Groups.Signals.XData = [0 20 20 1000]
      | sbobj.Groups.Signals.YData = [0 0 1 1]
      | sbobj.Groups.TimeRange = [0 1000]
  SWITCH : Outport  Tag=STV Outport
  wires:
  FromWs/1 -> Demux/1
  Demux/1 -> SWITCH/1

== system FireFighter_original/FF_Signals2/Environment1 ==
  note: F_hill
  note: F_eng_resistance
  note: F_resistance
  note: F_eng
  note: position
  note: speed
  note: slope
  gas : Inport
  brake : Inport  Port=2
  1/mass2 : Gain  Gain=0.001
  Discrete-Time Integrator : DiscreteIntegrator  SampleTime=-1  ICPrevOutput=DiscIntNeverNeededParam  ICPrevScaledInput=DiscIntNeverNeededParam
  Discrete-Time Integrator1 : DiscreteIntegrator  SampleTime=-1  ICPrevOutput=DiscIntNeverNeededParam  ICPrevScaledInput=DiscIntNeverNeededParam
  Fast - to - Slow : RateTransition  OutPortSampleTimeMultiple=0.05  OutPortSampleTime=0.1
  "Fast - to - Slow1 " : RateTransition  OutPortSampleTimeMultiple=0.05  OutPortSampleTime=0.1
  Fcn : Fcn  Expr=u(1)/0.005
  Gain1 : Gain  Gain=0.0005
  Max Torque by rpm6 : Lookup_n-D  NumberOfTableDimensions=1  BreakpointsForDimension1=[0;8;20;28;40;60;80;100;120;140;160;180;200]  Table=[165;180;180;170;170;150;115;97;80;70;60;50;40]  RndMeth=Simplest  InputSameDT=on
  Max Torque by rpm9 : Lookup_n-D  NumberOfTableDimensions=1  BreakpointsForDimension1=[0:1000:15000]  Table=[0;pi/60;pi/30;pi/20;pi/15;pi/12;0;0;-pi/18;-pi/36;0;0;0;0;0;0]  RndMeth=Simplest  InputSameDT=on
  Product1 : Product  RndMeth=Zero
  Scope{2..3,6..15,27} (13 alike) : Scope
      Scope10 settings: SaveName=ScopeData23
      Scope11 settings: TimeRange=10  YMin=-50  YMax=300  SaveName=ScopeData26
      Scope12 settings: SaveName=ScopeData32
      Scope13 settings: SaveName=ScopeData33
      Scope14 settings: SaveName=ScopeData15
      Scope15 settings: SaveName=ScopeData19
      Scope2 settings: TimeRange=10  YMin=-50  YMax=300  SaveName=ScopeData6
      Scope27 settings: TimeRange=10  YMin=-50  YMax=300  SaveName=ScopeData49
      Scope3 settings: SaveName=ScopeData8
      Scope6 settings: TimeRange=100  YMin=89.9904  YMax=89.9913  SaveName=ScopeData16
      Scope7 settings: SaveName=ScopeData10
      Scope8 settings: SaveName=ScopeData21
      Scope9 settings: SaveName=ScopeData22
  Slow - to - Fast : RateTransition  OutPortSampleTimeMultiple=0.05  OutPortSampleTime=0.05
  Step1 : Step  Time=0  After=1000
  Sum1 : Sum  Inputs=|++
  Sum4 : Sum  Inputs=|+---
  Trigonometric Function1 : Trigonometry
  brake force1 : Gain  Gain=10000
  g1 : Gain  Gain=9.80665
  mass3 : Gain  Gain=1000
  pos : Outport
  wires:
  Step1/1 -> Sum1/2
  Product1/1 -> Fcn/1
  brake force1/1 -> Scope12/1, Sum4/2
  Sum4/1 -> Scope7/1, 1/mass2/1
  1/mass2/1 -> Discrete-Time Integrator/1, Scope8/1
  Gain1/1 -> Scope13/1, Sum4/3
  gas/1 -> Scope14/1, Fast - to - Slow/1
  brake/1 -> Scope15/1, "Fast - to - Slow1 "/1
  Discrete-Time Integrator/1 -> Max Torque by rpm6/1, Gain1/1, Discrete-Time Integrator1/1, Scope6/1
  Discrete-Time Integrator1/1 -> Max Torque by rpm9/1, Scope2/1, Sum1/1
  Max Torque by rpm9/1 -> Trigonometric Function1/1
  g1/1 -> mass3/1
  Trigonometric Function1/1 -> g1/1
  mass3/1 -> Sum4/4, Scope3/1
  Fcn/1 -> Scope10/1, Sum4/1
  Fast - to - Slow/1 -> Product1/2
  "Fast - to - Slow1 "/1 -> brake force1/1
  Sum1/1 -> Scope27/1, Slow - to - Fast/1
  Slow - to - Fast/1 -> pos/1, Scope11/1
  Max Torque by rpm6/1 -> Product1/1, Scope9/1

== system FireFighter_original/FF_Signals2/FireFighter1 ==
  note: current speed
  note: speed=90
  pos : Inport
  Constant : Constant  Value=0
  Constant2 : Constant  Value=90
  Discrete Derivative : simulink/Discrete/Discrete Derivative  gainval=1.0  ICPrevScaledInput=0.0  InputProcessing=Inherited  OutMin=[]  OutMax=[]  OutDataType=fixdt(1, 16)  OutScaling=2^-10  DoSatur=off
  Discrete PID Controller : simulink/Continuous/PID Controller  Controller=PI  TimeDomain=Discrete-time  SampleTime=-1  IntegratorMethod=Forward Euler  FilterMethod=Forward Euler  Form=Parallel  P=0.05  I=0.000228325  D=0  N=100  InitialConditionSource=internal  InitialConditionForIntegrator=0  InitialConditionForFilter=0  ExternalReset=none  LimitOutput=on  UpperSaturationLimit=1  LowerSaturationLimit=-1  LinearizeAsGain=off  AntiWindupMode=back-calculation  Kb=0.01  TrackingMode=off  Kt=1  PParamMin=[]  PParamMax=[]  IParamMin=[]  IParamMax=[]  DParamMin=[]  DParamMax=[]  NParamMin=[]  NParamMax=[]  KbParamMin=[]  KbParamMax=[]  KtParamMin=[]  KtParamMax=[]  POutMin=[]  POutMax=[]  IOutMin=[]  IOutMax=[]  DOutMin=[]  DOutMax=[]  NOutMin=[]  NOutMax=[]  KbOutMin=[]  KbOutMax=[]  KtOutMin=[]  KtOutMax=[]  IntegratorOutMin=[]  IntegratorOutMax=[]  FilterOutMin=[]  FilterOutMax=[]  SumOutMin=[]  SumOutMax=[]  SumI1OutMin=[]  SumI1OutMax=[]  SumI2OutMin=[]  SumI2OutMax=[]  SumI3OutMin=[]  SumI3OutMax=[]  SumDOutMin=[]  SumDOutMax=[]  SaturationOutMin=[]  SaturationOutMax=[]  IntegratorContinuousStateAttributes=''  IntegratorStateMustResolveToSignalObject=off  IntegratorRTWStateStorageClass=Auto  FilterContinuousStateAttributes=''  FilterStateMustResolveToSignalObject=off  FilterRTWStateStorageClass=Auto
  Fast - to -Slow : RateTransition  OutPortSampleTimeMultiple=0.05  OutPortSampleTime=0.1
  Gain : Gain  Gain=50
  Gain1 : Gain  Gain=-1
  Scope{1..2,4..9,11..13} (11 alike) : Scope
      Scope1 settings: TimeRange=100  YMin=90  YMax=130
      Scope11 settings: YMin=-300  YMax=300  SaveName=ScopeData28
      Scope12 settings: YMin=-300  YMax=300  SaveName=ScopeData30
      Scope13 settings: SaveName=ScopeData31
      Scope2 settings: YMin=-300  YMax=300  SaveName=ScopeData2
      Scope4 settings: YMin=-300  YMax=300  SaveName=ScopeData17
      Scope5 settings: SaveName=ScopeData20
      Scope6 settings: YMin=-300  YMax=300  SaveName=ScopeData18
      Scope7 settings: YMin=-300  YMax=300  SaveName=ScopeData24
      Scope8 settings: TimeRange=10  SaveName=ScopeData25
      Scope9 settings: SaveName=ScopeData38
  Signal Builder : Subsystem  Tag=STV Subsys  LoadFcn=sigbuilder_block('load');  StartFcn=sigbuilder_block('start');  StopFcn=sigbuilder_block('stop');  ClipboardFcn=sigbuilder_block('clipboard');  mask(Sigbuilder block){}
      mask help: Simulink:masks:SigbuilderBlock_MD
      mask init:
      | if ~strcmp(get_param(bdroot(gcbh),'SimulationStatus'),'stopped') tuvar = sigbuilder_block('maskInit'); end
      settings: CopyFcn=sigbuilder_block('copy');  DeleteFcn=sigbuilder_block('delete');  ModelCloseFcn=sigbuilder_block('modelClose');  PreSaveFcn=sigbuilder_block('preSave');  PauseFcn=sigbuilder_block('pause');  ContinueFcn=sigbuilder_block('continue');  NameChangeFcn=sigbuilder_block('namechange');  OpenFcn=sigbuilder_block('open',[359.25 300.75 550.5 399.75 ]);  CloseFcn=sigbuilder_block('close');
      mask Display: plot(0, 0, 100, 100,[2, 2, 32, 32, 2], [68, 8, 8, 68, 68],[32, 2], [38, 38], [32, 19, 2],[53, 60, 44], [32, 17, 17, 2],[16, 16, 31, 31]);txt = getActiveGroup(gcbh);text(2, 100, txt,'verticalAlignment', 'top');
  Slow - to - Fast : RateTransition  OutPortSampleTimeMultiple=0.05  OutPortSampleTime=0.05
  Slow - to - Fast1 : RateTransition  OutPortSampleTimeMultiple=0.05  OutPortSampleTime=0.05
  Sum : Sum  Inputs=|+-
  Sum1 : Sum  Inputs=|++
  Switch : Switch
  Switch1 : Switch
  Zero-Order Hold : ZeroOrderHold  SampleTime=0.1
  gas : Outport
  brake : Outport  Port=2
  wires:
  Discrete Derivative/1 -> Scope8/1, Sum/2
  Signal Builder/1(Signal 1) -> Gain/1
  Gain/1 -> Zero-Order Hold/1
  Constant2/1 -> Sum1/2
  Discrete PID Controller/1 -> Scope2/1, Scope7/1, Switch/1, Switch/2, Switch1/2, Gain1/1
  Gain1/1 -> Switch1/3
  Switch/1 -> Slow - to - Fast/1, Scope4/1
  Constant/1 -> Switch/3, Switch1/1
  Switch1/1 -> Slow - to - Fast1/1, Scope6/1
  pos/1 -> Scope13/1, Fast - to -Slow/1
  Sum/1 -> Discrete PID Controller/1, Scope9/1
  Fast - to -Slow/1 -> Discrete Derivative/1, Scope5/1
  Slow - to - Fast/1 -> Scope11/1, gas/1
  Slow - to - Fast1/1 -> Scope12/1, brake/1
  Sum1/1 -> Scope1/1, Sum/1
  Zero-Order Hold/1 -> Sum1/1

== system FireFighter_original/FF_Signals2/Inaccuracy ==
  note: max
  pos_init : Inport
  hold : Inport  Port=2
  Mux29 : Mux  Inputs=2
  Product : Product
  Product1 : Product
  Scope{1..3,5..7,9} (7 alike) : Scope
      Scope1 settings: SaveName=ScopeData29
      Scope2 settings: SaveName=ScopeData43
      Scope3 settings: SaveName=ScopeData35
      Scope5 settings: SaveName=ScopeData46
      Scope6 settings: SaveName=ScopeData48
      Scope7 settings: TimeRange=150  SaveName=ScopeData57
      Scope9 settings: SaveName=ScopeData44
  Subsystem1 : Subsystem
  Subsystem2 : Subsystem
  Subtract1 : Sum  Inputs=-+
  result : Outport
  wires:
  Subsystem2/1(min) -> Product/1, Scope2/1  "min"
  pos_init/1 -> Subsystem1/1(pos_init), Subsystem2/1(pos_init), Scope1/1
  Mux29/1 -> result/1
  Subsystem1/1(max) -> Product1/2, Scope9/1
  Product/1 -> Mux29/1, Scope6/1, Subtract1/1
  Product1/1 -> Scope5/1, Mux29/2, Subtract1/2
  hold/1 -> Subsystem2/2(hold), Scope3/1, Product/2, Product1/1, Subsystem1/2(hold)
  Subtract1/1 -> Scope7/1

== system FireFighter_original/FF_Signals2/Inaccuracy1 ==
  note: max
  Hpos_inits : Inport
  holds : Inport  Port=2
  Mux29 : Mux  Inputs=2
  Product : Product
  Product1 : Product
  Scope{1..3,5..7,9} (7 alike) : Scope
      Scope1 settings: SaveName=ScopeData29
      Scope2 settings: SaveName=ScopeData43
      Scope3 settings: SaveName=ScopeData35
      Scope5 settings: SaveName=ScopeData46
      Scope6 settings: SaveName=ScopeData48
      Scope7 settings: TimeRange=150  SaveName=ScopeData57
      Scope9 settings: SaveName=ScopeData44
  Subsystem1 : Subsystem
  Subsystem2 : Subsystem
  Subtract1 : Sum  Inputs=-+
  result : Outport
  wires:
  Subsystem2/1(min) -> Product/1, Scope2/1  "min"
  Hpos_inits/1 -> Subsystem1/1(pos_init), Subsystem2/1(pos_init), Scope1/1
  Mux29/1 -> result/1
  Subsystem1/1(max) -> Product1/2, Scope9/1
  Product/1 -> Mux29/1, Scope6/1, Subtract1/1
  Product1/1 -> Scope5/1, Mux29/2, Subtract1/2
  holds/1 -> Subsystem2/2(hold), Scope3/1, Product/2, Product1/1, Subsystem1/2(hold)
  Subtract1/1 -> Scope7/1

== system FireFighter_original/FF_Signals2/Inaccuracy2 ==
  note: max
  Hpos_inits : Inport
  holds : Inport  Port=2
  Mux29 : Mux  Inputs=2
  Product : Product
  Product1 : Product
  Scope{1..3,5..7,9} (7 alike) : Scope
      Scope1 settings: SaveName=ScopeData29
      Scope2 settings: SaveName=ScopeData43
      Scope3 settings: SaveName=ScopeData35
      Scope5 settings: SaveName=ScopeData46
      Scope6 settings: SaveName=ScopeData48
      Scope7 settings: TimeRange=150  SaveName=ScopeData57
      Scope9 settings: SaveName=ScopeData44
  Subsystem1 : Subsystem
  Subsystem2 : Subsystem
  Subtract1 : Sum  Inputs=-+
  result : Outport
  wires:
  Subsystem2/1(min) -> Product/1, Scope2/1  "min"
  Hpos_inits/1 -> Subsystem1/1(pos_init), Subsystem2/1(pos_init), Scope1/1
  Mux29/1 -> result/1
  Subsystem1/1(max) -> Product1/2, Scope9/1
  Product/1 -> Mux29/1, Scope6/1, Subtract1/1
  Product1/1 -> Scope5/1, Mux29/2, Subtract1/2
  holds/1 -> Subsystem2/2(hold), Scope3/1, Product/2, Product1/1, Subsystem1/2(hold)
  Subtract1/1 -> Scope7/1

== system FireFighter_original/FF_Signals2/START THE MESSION2 ==
  Demux : Demux  Tag=STV Demux  Outputs=1
  FromWs : FromWorkspace  Tag=STV FromWs  VariableName=tuvar  SampleTime=0
      SigBuilderData=|
      | common.afterFinalStr = 'Extrapolate'
      | common.sampleTime = 0
      | dataSet.timeRange = [0 1000]
      | dataSet.name = 'Group 1'
      | sbobj.Groups.Name = 'Group 1'
      | sbobj.Groups.Signals.Name = 'SWITCH'
      | sbobj.Groups.Signals.XData = [0 20 20 1000]
      | sbobj.Groups.Signals.YData = [0 0 1 1]
      | sbobj.Groups.TimeRange = [0 1000]
  SWITCH : Outport  Tag=STV Outport
  wires:
  FromWs/1 -> Demux/1
  Demux/1 -> SWITCH/1
